simulink model "MassSpringDamper2018a"  (R2018a)
settings: Solver=FixedStepAuto  StartTime=0.0  StopTime=10  FixedStep=0.1  RelTol=1e-3
undefined symbols (not defined in the file): c, f, k, m
settings Model: Creator=ilab  LastModifiedBy=ilab
settings DebuggingCC: LibraryContextMissingDiagnostic=warning
settings SFSimCC: SimUseLocalCustomCode=on
settings RTWCC: RTWUseLocalCustomCode=on

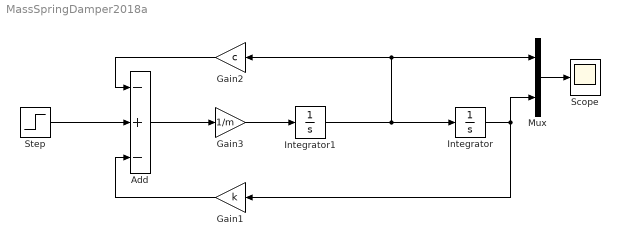
== system MassSpringDamper2018a ==
  Add : Sum  Inputs=-+-
  Gain1 : Gain  Gain=k
  Gain2 : Gain  Gain=c
  Gain3 : Gain  Gain=1/m
  Integrator : Integrator
  Integrator1 : Integrator
  Mux : Mux  Inputs=2
  Scope : Scope
  Step : Step  After=f  SampleTime=0
  wires:
  Integrator1/1 -> Integrator/1, Gain2/1, Mux/1
  Step/1 -> Add/2
  Add/1 -> Gain3/1
  Gain2/1 -> Add/1
  Gain1/1 -> Add/3
  Gain3/1 -> Integrator1/1
  Integrator/1 -> Mux/2, Gain1/1
  Mux/1 -> Scope/1
